simulink model "RTLDEMO (1)"  (R2023b)
settings: Solver=VariableStepAuto  StartTime=0.0  StopTime=10.0  RelTol=1e-3
undefined symbols (not defined in the file): startfcn_spectrum_analyzer
libraries: dspmlti4 x4, rtlsdr_book_library x2, sdrrlib x1, dspsrcs4 x1, dspobslib x1
settings Model: Creator=Mercedes  LastModifiedBy=Mercedes

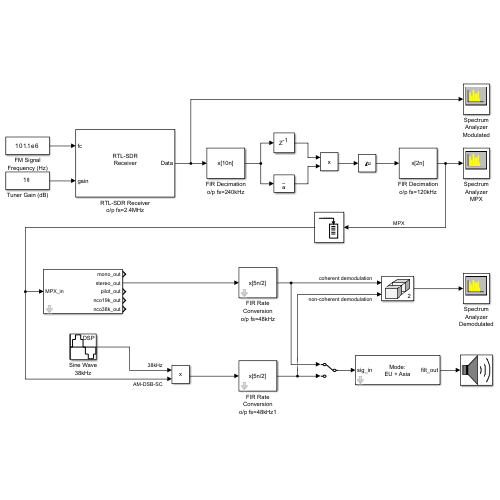
[thumbnail: Simulink's stored preview of the top-level diagram]
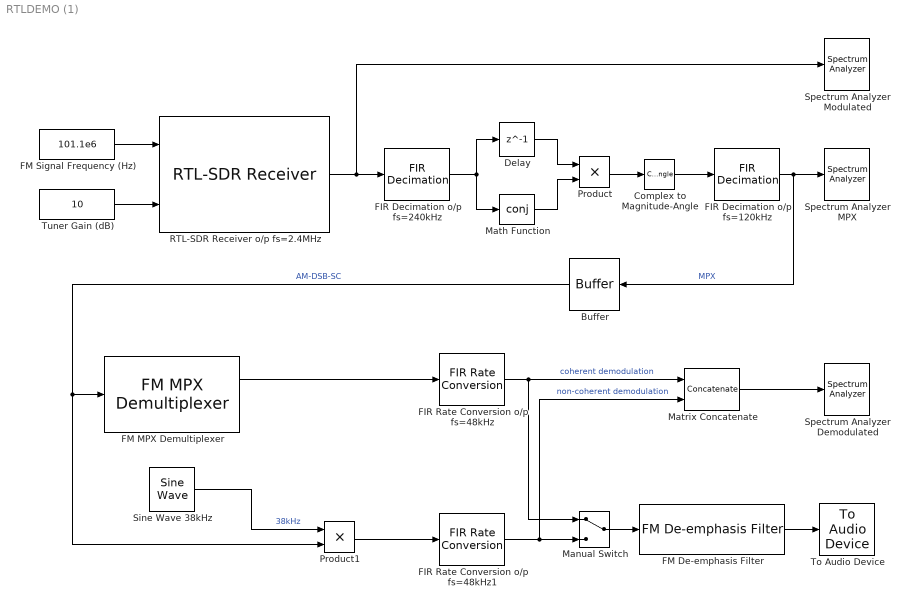
== system RTLDEMO (1) ==
  Buffer : Buffer  N=4000
  Complex to Magnitude-Angle : ComplexToMagnitudeAngle  Output=Angle
  Delay : Delay  DelayLength=1  InitialCondition=0  InputProcessing=Columns as channels (frame based)
  FIR Decimation o/p fs=120kHz : dspmlti4/FIR Decimation  FilterSource=Dialog parameters  h=firpm(100, [0 53e3 60e3 (240e3/2)]/(240e3/2), [1 1 0 0], [1 1],20)  D=2  filtStruct=Direct form  FilterObject=Hm_firdecim  InputProcessing=Columns as channels (frame based)  framing=Allow multirate processing  AllowArbitraryInputLength=off  inputOffset=0  outputBufInitCond=0  roundingMode=Floor  overflowMode=off  firstCoeffDataTypeStr=Inherit: Same word length as input  firstCoeffMin=[]  firstCoeffMax=[]  firstCoeffLastDataTypeStr=Inherit: Same word length as input  outputDataTypeStr=Inherit: Same as accumulator  outputMin=[]  outputMax=[]  outputLastDataTypeStr=Inherit: Same as accumulator
  FIR Decimation o/p fs=240kHz : dspmlti4/FIR Decimation  FilterSource=Dialog parameters  h=firpm(50, [0 120e3 240e3 (2.4e6/2)]/(2.4e6/2), [1 1 0 0], [1 1],20)  D=10  filtStruct=Direct form  FilterObject=Hm_firdecim  InputProcessing=Columns as channels (frame based)  framing=Allow multirate processing  AllowArbitraryInputLength=off  inputOffset=0  outputBufInitCond=0  roundingMode=Floor  overflowMode=off  firstCoeffDataTypeStr=Inherit: Same word length as input  firstCoeffMin=[]  firstCoeffMax=[]  firstCoeffLastDataTypeStr=Inherit: Same word length as input  outputDataTypeStr=Inherit: Same as accumulator  outputMin=[]  outputMax=[]  outputLastDataTypeStr=Inherit: Same as accumulator
  FIR Rate Conversion o/p fs=48kHz : dspmlti4/FIR Rate Conversion  FilterSource=Dialog parameters  L=2  h=firpm(100, [0 15e3 20e3 240e3/2]/(240e3/2), [1 1 0 0], [1 1],20)  M=5  FilterObject=Hm_firsrc  rateMode=Enforce single-rate processing  AllowArbitraryInputLength=off  roundingMode=Floor  overflowMode=off  firstCoeffDataTypeStr=Inherit: Same word length as input  firstCoeffMin=[]  firstCoeffMax=[]  firstCoeffLastDataTypeStr=Inherit: Same word length as input  outputDataTypeStr=Inherit: Same as accumulator  outputMin=[]  outputMax=[]  outputLastDataTypeStr=Inherit: Same as accumulator
  FIR Rate Conversion o/p fs=48kHz1 : dspmlti4/FIR Rate Conversion  FilterSource=Dialog parameters  L=2  h=firpm(100, [0 15e3 20e3 240e3/2]/(240e3/2), [1 1 0 0], [1 1],20)  M=5  FilterObject=Hm_firsrc  rateMode=Enforce single-rate processing  AllowArbitraryInputLength=off  roundingMode=Floor  overflowMode=off  firstCoeffDataTypeStr=Inherit: Same word length as input  firstCoeffMin=[]  firstCoeffMax=[]  firstCoeffLastDataTypeStr=Inherit: Same word length as input  outputDataTypeStr=Inherit: Same as accumulator  outputMin=[]  outputMax=[]  outputLastDataTypeStr=Inherit: Same as accumulator
  FM De-emphasis Filter : rtlsdr_book_library/FM Demod Tools/FM De-emphasis Filter  region=Europe, Asia  fs=48e3
      settings: SourceProductName=RTL-SDR Book Library
  FM MPX Demultiplexer : rtlsdr_book_library/FM Demod Tools/FM MPX Demultiplexer  fs=120e3  fq=19e3  Kpd=3  Kphe=2  frm_size=4000
      settings: SourceProductName=RTL-SDR Book Library
  FM Signal Frequency (Hz) : Constant  Value=101.1e6
  Manual Switch : ManualSwitch
  Math Function : Math  Operator=conj  SignedPower=on
  Matrix Concatenate : Concatenate  Mode=Multidimensional array  ConcatenateDimension=2
  Product : Product
  Product1 : Product  OutDataTypeStr=double
  RTL-SDR Receiver o/p fs=2.4MHz : sdrrlib/RTL-SDR Receiver  IPAddress=0  CenterFrequencySource=Input port  CenterFrequency=100e6  GainSource=Input port  Gain=25  ADCRate=2.4e6  FrequencyCorrection=0  LostSamplesOutputPort=off  LatencyOutputPort=off  OutputDataType=single  FrameLength=4096  EnableBurstMode=off  NumFramesInBurst=20  sobjType=sdrr.internal.SDRRTLReceiverSL  dataUDPPort=-1  ctrlUDPPort=-1  subDeviceList=nosubdev  sdrBlockType=SDRBlockTypeSLT.SDRRxBlock  requester=UNUSED_BY_SFCN  sdrExecutionMode=SDRExecutionModeSLT.ExecModeHW  BypassUserLogic=off  DecimatorSelect=DDC decimator  SourceSelect=RF data  SineAmplitude=16000  EnableInternalClock=off  BypassIQBalance=off  IFBandwidth=40e6  ADCRateSource=Dialog  IntermediateFrequency=0  DecimationFactorSource=Dialog  DecimationFactor=512  RFFrequencyIsTunable=logical(1)  SampleTime=(4096)/(2.4e6)  IFBandwidthSource=Dialog  SineFrequency=30000  BypassDCBlockingFilter=off  IntermediateFrequencySource=Dialog  IQBalanceCoefficients=64  SkipAllHardwareResetAndInitialization=off  EnableIQCalibrationTable=on  CacheIQCalibrationTable=off  EnableOffsetTuning=off  EnableRTLAGC=off  EnableTestMode=off  EnableTunerAGC=off  FrequencyCorrectionSource=Dialog  NumMLBuffers=128  NumUSBBuffers=16  RTLCrystalFrequency=28800000  TunerCrystalFrequency=28800000
  Sine Wave 38kHz : dspsrcs4/Sine Wave  Amplitude=2  Frequency=38e3  Phase=0  SampleMode=Discrete  OutComplex=Real  CompMethod=Trigonometric fcn  TableSize=Speed  SampleTime=1/120e3  SamplesPerFrame=4000  ResetState=Restart at time zero  OutputFrames=on  dataType=single  wordLen=16  udDataType=sfix(16)  fracBitsMode=Best precision  numFracBits=15  OutDataTypeStr=single  LastOutDataTypeStr=single
  Spectrum Analyzer Demodulated : SpectrumAnalyzer  StartFcn=startfcn_spectrum_analyzer;  WindowPosition=[1084.000000,622.000000,778.000000,262.000000,]  Visible=on  ScopeFrameLocation=window  Method=Welch  SampleRate=48000  AxesScaling=Manual  Span=400000  StartFrequency=-200000  StopFrequency=200000  AveragingMethod=Running  YLabel=dBm  YLimits=[-90,25]  ColorLimits=[-145.27268916534743,20]  ShowGrid=off  ShowLegend=on  DefaultConfigurationName=spbscopes.SpectrumAnalyzerBlockCfg
  Spectrum Analyzer MPX : SpectrumAnalyzer  StartFcn=startfcn_spectrum_analyzer;  WindowPosition=[1085.000000,370.000000,778.000000,262.000000,]  Visible=on  ScopeFrameLocation=window  Method=Welch  SampleRate=120000  AxesScaling=Manual  Span=400000  StartFrequency=-200000  StopFrequency=200000  AveragingMethod=Running  YLabel=dBm  ColorLimits=[-145.27268916534743,20]  ShowGrid=off  DefaultConfigurationName=spbscopes.SpectrumAnalyzerBlockCfg
  Spectrum Analyzer Modulated : SpectrumAnalyzer  StartFcn=startfcn_spectrum_analyzer;  WindowPosition=[1085.000000,171.000000,778.000000,225.000000,]  Visible=on  ScopeFrameLocation=window  Method=Welch  SampleRate=240000  AxesScaling=Manual  Span=400000  StartFrequency=-200000  StopFrequency=200000  AveragingMethod=Running  YLabel=dBm  YLimits=[-69.383930992470468,32.02048051388072]  ColorLimits=[-145.27268916534743,20]  ShowGrid=off  DefaultConfigurationName=spbscopes.SpectrumAnalyzerBlockCfg
  To Audio Device : dspobslib/To Audio Device  deviceName=Default  inheritSampleRate=on  sampleRate=44100  deviceDatatype=Determine from input data type  autoBufferSize=on  bufferSize=4096  queueDuration=1.0  defaultOutputChannelMapping=on  outputChannelMapping=1  outputNumUnderrunSamples=off
  Tuner Gain (dB) : Constant  Value=10
  wires:
  FM Signal Frequency (Hz)/1 -> RTL-SDR Receiver o/p fs=2.4MHz/1
  Manual Switch/1 -> FM De-emphasis Filter/1
  Matrix Concatenate/1 -> Spectrum Analyzer Demodulated/1
  Tuner Gain (dB)/1 -> RTL-SDR Receiver o/p fs=2.4MHz/2
  Complex to Magnitude-Angle/1 -> FIR Decimation o/p fs=120kHz/1
  FM De-emphasis Filter/1 -> To Audio Device/1
  FIR Rate Conversion o/p fs=48kHz1/1 -> Matrix Concatenate/2, Manual Switch/2  "non-coherent demodulation"
  RTL-SDR Receiver o/p fs=2.4MHz/1 -> Spectrum Analyzer Modulated/1, FIR Decimation o/p fs=240kHz/1
  FIR Rate Conversion o/p fs=48kHz/1 -> Manual Switch/1, Matrix Concatenate/1  "coherent demodulation"
  Product1/1 -> FIR Rate Conversion o/p fs=48kHz1/1
  FIR Decimation o/p fs=120kHz/1 -> Spectrum Analyzer MPX/1, Buffer/1  "MPX"
  Product/1 -> Complex to Magnitude-Angle/1
  FIR Decimation o/p fs=240kHz/1 -> Delay/1, Math Function/1
  Sine Wave 38kHz/1 -> Product1/1  "38kHz"
  Math Function/1 -> Product/2
  Buffer/1 -> Product1/2, FM MPX Demultiplexer/1  "AM-DSB-SC"
  Delay/1 -> Product/1
  FM MPX Demultiplexer/2 -> FIR Rate Conversion o/p fs=48kHz/1
